simulink model "dsp_blr_hikaku_nakamura_futagi"  (R2018a)
settings: Solver=VariableStepAuto  StartTime=0.0  StopTime=100e-6  RelTol=1e-3
values from neighbouring files (symbols this model uses):
  BASELINE = 0    [dsp_blr.mat]
libraries: xbsIndex_r4 x934, xrbsSSR_Library x35, simulink x3, dspsigattribs x2, hdlsllib x2
(part 4 of 6)

== system dsp_blr_hikaku_nakamura_futagi/8sample_average 1/Vector_sum ==
  tdata_in : Inport
  AddSub{,1..3} (4 alike) : xbsIndex_r4/AddSub  mode=Addition  use_carryin=off  use_carryout=off  en=off  latency=0  precision=User Defined  arith_type="Signed  (2's comp)"  n_bits=17  bin_pt=4  quantization=Truncate  overflow=Wrap  use_behavioral_HDL=off  hw_selection=Fabric  pipelined=off  dbl_ovrd=off  block_type=addsub
  AddSub4 : xbsIndex_r4/AddSub  mode=Addition  use_carryin=off  use_carryout=off  en=off  latency=0  precision=Full  arith_type="Signed  (2's comp)"  n_bits=18  bin_pt=4  quantization=Truncate  overflow=Wrap  use_behavioral_HDL=off  hw_selection=Fabric  pipelined=off  dbl_ovrd=off  block_type=addsub
  AddSub5 : xbsIndex_r4/AddSub  mode=Addition  use_carryin=off  use_carryout=off  en=off  latency=0  precision=Full  arith_type="Signed  (2's comp)"  n_bits=18  bin_pt=4  quantization=Truncate  overflow=Wrap  use_behavioral_HDL=off  hw_selection=Fabric  pipelined=off  dbl_ovrd=off  block_type=addsub
  AddSub6 : xbsIndex_r4/AddSub  mode=Addition  use_carryin=off  use_carryout=off  en=off  latency=0  precision=User Defined  arith_type="Signed  (2's comp)"  n_bits=19  bin_pt=4  quantization=Truncate  overflow=Wrap  use_behavioral_HDL=off  hw_selection=Fabric  pipelined=off  dbl_ovrd=off  block_type=addsub
  Reinterpret{,1..7} (8 alike) : xbsIndex_r4/Reinterpret  force_arith_type=on  arith_type="Signed  (2's comp)"  force_bin_pt=on  bin_pt=4  block_type=reinterpret
  Slice : xbsIndex_r4/Slice  nbits=16  boolean_output=off  mode=Two Bit Locations  bit1=15  base1=LSB of Input  bit0=0  base0=LSB of Input  dbl_ovrd=off  block_type=slice
  Slice1 : xbsIndex_r4/Slice  nbits=16  boolean_output=off  mode=Two Bit Locations  bit1=31  base1=LSB of Input  bit0=16  base0=LSB of Input  dbl_ovrd=off  block_type=slice
  Slice2 : xbsIndex_r4/Slice  nbits=16  boolean_output=off  mode=Two Bit Locations  bit1=47  base1=LSB of Input  bit0=32  base0=LSB of Input  dbl_ovrd=off  block_type=slice
  Slice3 : xbsIndex_r4/Slice  nbits=16  boolean_output=off  mode=Two Bit Locations  bit1=63  base1=LSB of Input  bit0=48  base0=LSB of Input  dbl_ovrd=off  block_type=slice
  Slice4 : xbsIndex_r4/Slice  nbits=16  boolean_output=off  mode=Two Bit Locations  bit1=79  base1=LSB of Input  bit0=64  base0=LSB of Input  dbl_ovrd=off  block_type=slice
  Slice5 : xbsIndex_r4/Slice  nbits=16  boolean_output=off  mode=Two Bit Locations  bit1=95  base1=LSB of Input  bit0=80  base0=LSB of Input  dbl_ovrd=off  block_type=slice
  Slice6 : xbsIndex_r4/Slice  nbits=16  boolean_output=off  mode=Two Bit Locations  bit1=111  base1=LSB of Input  bit0=96  base0=LSB of Input  dbl_ovrd=off  block_type=slice
  Slice7 : xbsIndex_r4/Slice  nbits=16  boolean_output=off  mode=Two Bit Locations  bit1=127  base1=LSB of Input  bit0=112  base0=LSB of Input  dbl_ovrd=off  block_type=slice
  Vector Reinterpret : xrbsSSR_Library/Vector Reinterpret  sg_ssr=8  sg_ssr_prev=8  force_arith_type=on  arith_type=Unsigned  force_bin_pt=on  bin_pt=0  block_type=reinterpret_ssr
      settings: SourceProductName=Xilinx SSR Blockset  infoedit="The Vector Reinterpret block Changes vector input signal type without altering the binary representation. You can change the signal between signed and unsigned, and relocate the binary point.<br><br>Hardware notes: In hardware this block costs nothing.<br><br>Example:  Suppose the input is 6 bits wide, signed, with 2 fractional bits, and the output is forced to unsigned with 0 fractional bits.  Then an input of -2.0 (1110.00 in binary 2's complement) becomes an output of 56 (111000 in binary)."
  Vector2Scalar : xrbsSSR_Library/Vector2Scalar  sg_ssr=8  sg_ssr_prev=8  sg_ssr_name=vect_Vector2Scalar  block_type=vector2scalar_ssr
      settings: SourceProductName=Xilinx SSR Blockset
  sum_data_out : Outport  OutDataTypeStr=fixdt(1,19,4)
  wires:
  AddSub4/1 -> AddSub6/1
  Vector2Scalar/1 -> Slice7/1, Slice6/1, Slice5/1, Slice4/1, Slice2/1, Slice/1, Slice1/1, Slice3/1
  AddSub1/1 -> AddSub4/2
  AddSub5/1 -> AddSub6/2
  AddSub/1 -> AddSub4/1
  AddSub3/1 -> AddSub5/2
  AddSub2/1 -> AddSub5/1
  AddSub6/1 -> sum_data_out/1
  Slice/1 -> Reinterpret/1
  Slice1/1 -> Reinterpret1/1
  Slice2/1 -> Reinterpret2/1
  Slice3/1 -> Reinterpret3/1
  Slice4/1 -> Reinterpret4/1
  Slice5/1 -> Reinterpret5/1
  Slice6/1 -> Reinterpret6/1
  Slice7/1 -> Reinterpret7/1
  Reinterpret/1 -> AddSub/1
  Reinterpret1/1 -> AddSub/2
  Reinterpret2/1 -> AddSub1/1
  Reinterpret3/1 -> AddSub1/2
  Reinterpret4/1 -> AddSub2/1
  Reinterpret5/1 -> AddSub2/2
  Reinterpret6/1 -> AddSub3/1
  Reinterpret7/1 -> AddSub3/2
  tdata_in/1 -> Vector Reinterpret/1
  Vector Reinterpret/1 -> Vector2Scalar/1

== system dsp_blr_hikaku_nakamura_futagi/8sample_average 1/scaling ==
  valid_in : Inport
  data_in : Inport  Port=2
  Shift : xbsIndex_r4/Shift  shift_dir=Right  shift_bits=3  en=off  latency=1  precision=Full  arith_type="Signed  (2's comp)"  n_bits=16  bin_pt=14  quantization=Truncate  overflow=Wrap  dbl_ovrd=off  block_type=shift
  tvalid_delay : xbsIndex_r4/Delay  rst=off  infoeditControl=Selection of Reset will increase slice count due to use of real FFs and instead of SRLs  en=off  latency=1  reg_retiming=off  dbl_ovrd=off  block_type=delay
  valid_out : Outport
  data_out : Outport  Port=2
  wires:
  valid_in/1 -> tvalid_delay/1
  tvalid_delay/1 -> valid_out/1
  data_in/1 -> Shift/1
  Shift/1 -> data_out/1

== system dsp_blr_hikaku_nakamura_futagi/8sample_average 3/Vector_sum ==
  tdata_in : Inport
  AddSub{,1..3} (4 alike) : xbsIndex_r4/AddSub  mode=Addition  use_carryin=off  use_carryout=off  en=off  latency=0  precision=User Defined  arith_type="Signed  (2's comp)"  n_bits=17  bin_pt=4  quantization=Truncate  overflow=Wrap  use_behavioral_HDL=off  hw_selection=Fabric  pipelined=off  dbl_ovrd=off  block_type=addsub
  AddSub4 : xbsIndex_r4/AddSub  mode=Addition  use_carryin=off  use_carryout=off  en=off  latency=0  precision=Full  arith_type="Signed  (2's comp)"  n_bits=18  bin_pt=4  quantization=Truncate  overflow=Wrap  use_behavioral_HDL=off  hw_selection=Fabric  pipelined=off  dbl_ovrd=off  block_type=addsub
  AddSub5 : xbsIndex_r4/AddSub  mode=Addition  use_carryin=off  use_carryout=off  en=off  latency=0  precision=Full  arith_type="Signed  (2's comp)"  n_bits=18  bin_pt=4  quantization=Truncate  overflow=Wrap  use_behavioral_HDL=off  hw_selection=Fabric  pipelined=off  dbl_ovrd=off  block_type=addsub
  AddSub6 : xbsIndex_r4/AddSub  mode=Addition  use_carryin=off  use_carryout=off  en=off  latency=0  precision=User Defined  arith_type="Signed  (2's comp)"  n_bits=19  bin_pt=4  quantization=Truncate  overflow=Wrap  use_behavioral_HDL=off  hw_selection=Fabric  pipelined=off  dbl_ovrd=off  block_type=addsub
  Gateway Out6 : xbsIndex_r4/Gateway Out  inherit_from_input=off  hdl_port=on  rows=1  columns=1  UseAsDAC=off  DACChannel='1'  interface=None  automatic_assignment=on  address_offset=hex2dec('00')  intf_name=''  intf_description=''  timing_constraint=None  locs_specified=off  LOCs={}  io_standard={}  block_type=gatewayout
  Reinterpret{,1..7} (8 alike) : xbsIndex_r4/Reinterpret  force_arith_type=on  arith_type="Signed  (2's comp)"  force_bin_pt=on  bin_pt=4  block_type=reinterpret
  Scope8 : Scope  NumInputPorts=2
  Slice : xbsIndex_r4/Slice  nbits=16  boolean_output=off  mode=Two Bit Locations  bit1=15  base1=LSB of Input  bit0=0  base0=LSB of Input  dbl_ovrd=off  block_type=slice
  Slice1 : xbsIndex_r4/Slice  nbits=16  boolean_output=off  mode=Two Bit Locations  bit1=31  base1=LSB of Input  bit0=16  base0=LSB of Input  dbl_ovrd=off  block_type=slice
  Slice2 : xbsIndex_r4/Slice  nbits=16  boolean_output=off  mode=Two Bit Locations  bit1=47  base1=LSB of Input  bit0=32  base0=LSB of Input  dbl_ovrd=off  block_type=slice
  Slice3 : xbsIndex_r4/Slice  nbits=16  boolean_output=off  mode=Two Bit Locations  bit1=63  base1=LSB of Input  bit0=48  base0=LSB of Input  dbl_ovrd=off  block_type=slice
  Slice4 : xbsIndex_r4/Slice  nbits=16  boolean_output=off  mode=Two Bit Locations  bit1=79  base1=LSB of Input  bit0=64  base0=LSB of Input  dbl_ovrd=off  block_type=slice
  Slice5 : xbsIndex_r4/Slice  nbits=16  boolean_output=off  mode=Two Bit Locations  bit1=95  base1=LSB of Input  bit0=80  base0=LSB of Input  dbl_ovrd=off  block_type=slice
  Slice6 : xbsIndex_r4/Slice  nbits=16  boolean_output=off  mode=Two Bit Locations  bit1=111  base1=LSB of Input  bit0=96  base0=LSB of Input  dbl_ovrd=off  block_type=slice
  Slice7 : xbsIndex_r4/Slice  nbits=16  boolean_output=off  mode=Two Bit Locations  bit1=127  base1=LSB of Input  bit0=112  base0=LSB of Input  dbl_ovrd=off  block_type=slice
  Vector Real Gateway Out1 : xrbsSSR_Library/Vector Real Gateway Out  inherit_from_input=off  hdl_port=on  rows=1  columns=1  UseAsDAC=off  DACChannel='1'  interface=None  automatic_assignment=on  address_offset=hex2dec('00')  intf_name=''  intf_description=''  timing_constraint=None  locs_specified=off  LOCs={}  io_standard={}  block_type=realgatewayout_ssr  sg_ssr=8  sg_ssr_prev=8  sg_ssr_name=vect_real_gwayout
      settings: SourceProductName=Xilinx SSR Blockset  infoedit=The Vector Real Gateway out block converts Xilinx fixed-point or floating-point type vector inputs into vector ouputs of type Simulink integer, single, double, or fixed-point.<br><br>Hardware notes: In hardware these blocks become top level output ports or are discarded, depending on how they are configured.
  Vector Reinterpret : xrbsSSR_Library/Vector Reinterpret  sg_ssr=8  sg_ssr_prev=8  force_arith_type=on  arith_type=Unsigned  force_bin_pt=on  bin_pt=0  block_type=reinterpret_ssr
      settings: SourceProductName=Xilinx SSR Blockset  infoedit="The Vector Reinterpret block Changes vector input signal type without altering the binary representation. You can change the signal between signed and unsigned, and relocate the binary point.<br><br>Hardware notes: In hardware this block costs nothing.<br><br>Example:  Suppose the input is 6 bits wide, signed, with 2 fractional bits, and the output is forced to unsigned with 0 fractional bits.  Then an input of -2.0 (1110.00 in binary 2's complement) becomes an output of 56 (111000 in binary)."
  Vector2Scalar : xrbsSSR_Library/Vector2Scalar  sg_ssr=8  sg_ssr_prev=8  sg_ssr_name=vect_Vector2Scalar  block_type=vector2scalar_ssr
      settings: SourceProductName=Xilinx SSR Blockset
  sum_data_out : Outport  OutDataTypeStr=fixdt(1,19,4)
  wires:
  AddSub4/1 -> AddSub6/1
  Vector2Scalar/1 -> Slice7/1, Slice6/1, Slice5/1, Slice4/1, Slice2/1, Slice/1, Slice1/1, Slice3/1
  AddSub1/1 -> AddSub4/2
  AddSub5/1 -> AddSub6/2
  AddSub/1 -> AddSub4/1
  AddSub3/1 -> AddSub5/2
  AddSub2/1 -> AddSub5/1
  AddSub6/1 -> Gateway Out6/1, sum_data_out/1
  Slice/1 -> Reinterpret/1
  Slice1/1 -> Reinterpret1/1
  Slice2/1 -> Reinterpret2/1
  Slice3/1 -> Reinterpret3/1
  Slice4/1 -> Reinterpret4/1
  Slice5/1 -> Reinterpret5/1
  Slice6/1 -> Reinterpret6/1
  Slice7/1 -> Reinterpret7/1
  Reinterpret/1 -> AddSub/1
  Reinterpret1/1 -> AddSub/2
  Reinterpret2/1 -> AddSub1/1
  Reinterpret3/1 -> AddSub1/2
  Reinterpret4/1 -> AddSub2/1
  Reinterpret5/1 -> AddSub2/2
  Reinterpret6/1 -> AddSub3/1
  Reinterpret7/1 -> AddSub3/2
  tdata_in/1 -> Vector Real Gateway Out1/1, Vector Reinterpret/1
  Vector Reinterpret/1 -> Vector2Scalar/1
  Gateway Out6/1 -> Scope8/2  "scalar"
  Vector Real Gateway Out1/1 -> Scope8/1  "vector"

== system dsp_blr_hikaku_nakamura_futagi/8sample_average 3/scaling ==
  valid_in : Inport
  data_in : Inport  Port=2
  Gateway Out1 : xbsIndex_r4/Gateway Out  inherit_from_input=off  hdl_port=on  rows=1  columns=1  UseAsDAC=off  DACChannel='1'  interface=None  automatic_assignment=on  address_offset=hex2dec('00')  intf_name=''  intf_description=''  timing_constraint=None  locs_specified=off  LOCs={}  io_standard={}  block_type=gatewayout
  Gateway Out6 : xbsIndex_r4/Gateway Out  inherit_from_input=off  hdl_port=on  rows=1  columns=1  UseAsDAC=off  DACChannel='1'  interface=None  automatic_assignment=on  address_offset=hex2dec('00')  intf_name=''  intf_description=''  timing_constraint=None  locs_specified=off  LOCs={}  io_standard={}  block_type=gatewayout
  Scope8 : Scope  NumInputPorts=2
  Shift : xbsIndex_r4/Shift  shift_dir=Right  shift_bits=3  en=off  latency=1  precision=Full  arith_type="Signed  (2's comp)"  n_bits=16  bin_pt=14  quantization=Truncate  overflow=Wrap  dbl_ovrd=off  block_type=shift
  tvalid_delay : xbsIndex_r4/Delay  rst=off  infoeditControl=Selection of Reset will increase slice count due to use of real FFs and instead of SRLs  en=off  latency=1  reg_retiming=off  dbl_ovrd=off  block_type=delay
  valid_out : Outport
  data_out : Outport  Port=2
  wires:
  valid_in/1 -> tvalid_delay/1
  tvalid_delay/1 -> valid_out/1
  data_in/1 -> Gateway Out1/1, Shift/1
  Gateway Out6/1 -> Scope8/2  "after"
  Gateway Out1/1 -> Scope8/1  "before"
  Shift/1 -> Gateway Out6/1, data_out/1

== system dsp_blr_hikaku_nakamura_futagi/Ave10/Subsystem1 ==
  In1 : Inport
  AddSub{,1,3,8..9,12} (6 alike) : xbsIndex_r4/AddSub  mode=Addition  use_carryin=off  use_carryout=off  en=off  latency=0  precision=User Defined  arith_type="Signed  (2's comp)"  n_bits=17  bin_pt=4  quantization=Truncate  overflow=Wrap  use_behavioral_HDL=off  hw_selection=Fabric  pipelined=off  dbl_ovrd=off  block_type=addsub
  AddSub4 : xbsIndex_r4/AddSub  mode=Addition  use_carryin=off  use_carryout=off  en=off  latency=0  precision=Full  arith_type="Signed  (2's comp)"  n_bits=18  bin_pt=4  quantization=Truncate  overflow=Wrap  use_behavioral_HDL=off  hw_selection=Fabric  pipelined=off  dbl_ovrd=off  block_type=addsub
  Delay1 : xbsIndex_r4/Delay  rst=off  infoeditControl=Selection of Reset will increase slice count due to use of real FFs and instead of SRLs  en=off  latency=1  reg_retiming=off  dbl_ovrd=off  block_type=delay
  Delay10 : xbsIndex_r4/Delay  rst=off  infoeditControl=Selection of Reset will increase slice count due to use of real FFs and instead of SRLs  en=off  latency=7  reg_retiming=off  dbl_ovrd=off  block_type=delay
  Delay2 : xbsIndex_r4/Delay  rst=off  infoeditControl=Selection of Reset will increase slice count due to use of real FFs and instead of SRLs  en=off  latency=2  reg_retiming=off  dbl_ovrd=off  block_type=delay
  Delay5 : xbsIndex_r4/Delay  rst=off  infoeditControl=Selection of Reset will increase slice count due to use of real FFs and instead of SRLs  en=off  latency=3  reg_retiming=off  dbl_ovrd=off  block_type=delay
  Delay7 : xbsIndex_r4/Delay  rst=off  infoeditControl=Selection of Reset will increase slice count due to use of real FFs and instead of SRLs  en=off  latency=4  reg_retiming=off  dbl_ovrd=off  block_type=delay
  Delay8 : xbsIndex_r4/Delay  rst=off  infoeditControl=Selection of Reset will increase slice count due to use of real FFs and instead of SRLs  en=off  latency=5  reg_retiming=off  dbl_ovrd=off  block_type=delay
  Delay9 : xbsIndex_r4/Delay  rst=off  infoeditControl=Selection of Reset will increase slice count due to use of real FFs and instead of SRLs  en=off  latency=6  reg_retiming=off  dbl_ovrd=off  block_type=delay
  Out1 : Outport
  wires:
  AddSub/1 -> AddSub1/1
  In1/1 -> AddSub/1, Delay10/1, Delay9/1, Delay8/1, Delay7/1, Delay5/1, Delay2/1, Delay1/1
  AddSub9/1 -> AddSub12/2
  Delay1/1 -> AddSub/2
  Delay10/1 -> AddSub9/2
  Delay9/1 -> AddSub9/1
  Delay2/1 -> AddSub3/1
  AddSub4/1 -> Out1/1
  Delay7/1 -> AddSub8/1
  AddSub1/1 -> AddSub4/1
  Delay8/1 -> AddSub8/2
  AddSub8/1 -> AddSub12/1
  Delay5/1 -> AddSub3/2
  AddSub3/1 -> AddSub1/2
  AddSub12/1 -> AddSub4/2

== system dsp_blr_hikaku_nakamura_futagi/Ave10/Subsystem2 ==
  In1 : Inport
  AddSub{,1,3,8..9,12} (6 alike) : xbsIndex_r4/AddSub  mode=Addition  use_carryin=off  use_carryout=off  en=off  latency=0  precision=User Defined  arith_type="Signed  (2's comp)"  n_bits=17  bin_pt=4  quantization=Truncate  overflow=Wrap  use_behavioral_HDL=off  hw_selection=Fabric  pipelined=off  dbl_ovrd=off  block_type=addsub
  AddSub4 : xbsIndex_r4/AddSub  mode=Addition  use_carryin=off  use_carryout=off  en=off  latency=0  precision=Full  arith_type="Signed  (2's comp)"  n_bits=18  bin_pt=4  quantization=Truncate  overflow=Wrap  use_behavioral_HDL=off  hw_selection=Fabric  pipelined=off  dbl_ovrd=off  block_type=addsub
  Delay1 : xbsIndex_r4/Delay  rst=off  infoeditControl=Selection of Reset will increase slice count due to use of real FFs and instead of SRLs  en=off  latency=1  reg_retiming=off  dbl_ovrd=off  block_type=delay
  Delay10 : xbsIndex_r4/Delay  rst=off  infoeditControl=Selection of Reset will increase slice count due to use of real FFs and instead of SRLs  en=off  latency=7  reg_retiming=off  dbl_ovrd=off  block_type=delay
  Delay2 : xbsIndex_r4/Delay  rst=off  infoeditControl=Selection of Reset will increase slice count due to use of real FFs and instead of SRLs  en=off  latency=2  reg_retiming=off  dbl_ovrd=off  block_type=delay
  Delay5 : xbsIndex_r4/Delay  rst=off  infoeditControl=Selection of Reset will increase slice count due to use of real FFs and instead of SRLs  en=off  latency=3  reg_retiming=off  dbl_ovrd=off  block_type=delay
  Delay7 : xbsIndex_r4/Delay  rst=off  infoeditControl=Selection of Reset will increase slice count due to use of real FFs and instead of SRLs  en=off  latency=4  reg_retiming=off  dbl_ovrd=off  block_type=delay
  Delay8 : xbsIndex_r4/Delay  rst=off  infoeditControl=Selection of Reset will increase slice count due to use of real FFs and instead of SRLs  en=off  latency=5  reg_retiming=off  dbl_ovrd=off  block_type=delay
  Delay9 : xbsIndex_r4/Delay  rst=off  infoeditControl=Selection of Reset will increase slice count due to use of real FFs and instead of SRLs  en=off  latency=6  reg_retiming=off  dbl_ovrd=off  block_type=delay
  Out1 : Outport
  wires:
  AddSub/1 -> AddSub1/1
  In1/1 -> AddSub/1, Delay10/1, Delay9/1, Delay8/1, Delay7/1, Delay5/1, Delay2/1, Delay1/1
  AddSub9/1 -> AddSub12/2
  Delay1/1 -> AddSub/2
  Delay10/1 -> AddSub9/2
  Delay9/1 -> AddSub9/1
  Delay2/1 -> AddSub3/1
  AddSub4/1 -> Out1/1
  Delay7/1 -> AddSub8/1
  AddSub1/1 -> AddSub4/1
  Delay8/1 -> AddSub8/2
  AddSub8/1 -> AddSub12/1
  Delay5/1 -> AddSub3/2
  AddSub3/1 -> AddSub1/2
  AddSub12/1 -> AddSub4/2

== system dsp_blr_hikaku_nakamura_futagi/Ave10/Subsystem3 ==
  In1 : Inport
  AddSub{,1,3,8..9,12} (6 alike) : xbsIndex_r4/AddSub  mode=Addition  use_carryin=off  use_carryout=off  en=off  latency=0  precision=User Defined  arith_type="Signed  (2's comp)"  n_bits=17  bin_pt=4  quantization=Truncate  overflow=Wrap  use_behavioral_HDL=off  hw_selection=Fabric  pipelined=off  dbl_ovrd=off  block_type=addsub
  AddSub4 : xbsIndex_r4/AddSub  mode=Addition  use_carryin=off  use_carryout=off  en=off  latency=0  precision=Full  arith_type="Signed  (2's comp)"  n_bits=18  bin_pt=4  quantization=Truncate  overflow=Wrap  use_behavioral_HDL=off  hw_selection=Fabric  pipelined=off  dbl_ovrd=off  block_type=addsub
  Delay1 : xbsIndex_r4/Delay  rst=off  infoeditControl=Selection of Reset will increase slice count due to use of real FFs and instead of SRLs  en=off  latency=1  reg_retiming=off  dbl_ovrd=off  block_type=delay
  Delay10 : xbsIndex_r4/Delay  rst=off  infoeditControl=Selection of Reset will increase slice count due to use of real FFs and instead of SRLs  en=off  latency=7  reg_retiming=off  dbl_ovrd=off  block_type=delay
  Delay2 : xbsIndex_r4/Delay  rst=off  infoeditControl=Selection of Reset will increase slice count due to use of real FFs and instead of SRLs  en=off  latency=2  reg_retiming=off  dbl_ovrd=off  block_type=delay
  Delay5 : xbsIndex_r4/Delay  rst=off  infoeditControl=Selection of Reset will increase slice count due to use of real FFs and instead of SRLs  en=off  latency=3  reg_retiming=off  dbl_ovrd=off  block_type=delay
  Delay7 : xbsIndex_r4/Delay  rst=off  infoeditControl=Selection of Reset will increase slice count due to use of real FFs and instead of SRLs  en=off  latency=4  reg_retiming=off  dbl_ovrd=off  block_type=delay
  Delay8 : xbsIndex_r4/Delay  rst=off  infoeditControl=Selection of Reset will increase slice count due to use of real FFs and instead of SRLs  en=off  latency=5  reg_retiming=off  dbl_ovrd=off  block_type=delay
  Delay9 : xbsIndex_r4/Delay  rst=off  infoeditControl=Selection of Reset will increase slice count due to use of real FFs and instead of SRLs  en=off  latency=6  reg_retiming=off  dbl_ovrd=off  block_type=delay
  Out1 : Outport
  wires:
  AddSub/1 -> AddSub1/1
  In1/1 -> AddSub/1, Delay10/1, Delay9/1, Delay8/1, Delay7/1, Delay5/1, Delay2/1, Delay1/1
  AddSub9/1 -> AddSub12/2
  Delay1/1 -> AddSub/2
  Delay10/1 -> AddSub9/2
  Delay9/1 -> AddSub9/1
  Delay2/1 -> AddSub3/1
  AddSub4/1 -> Out1/1
  Delay7/1 -> AddSub8/1
  AddSub1/1 -> AddSub4/1
  Delay8/1 -> AddSub8/2
  AddSub8/1 -> AddSub12/1
  Delay5/1 -> AddSub3/2
  AddSub3/1 -> AddSub1/2
  AddSub12/1 -> AddSub4/2

== system dsp_blr_hikaku_nakamura_futagi/Ave10/Subsystem4 ==
  In1 : Inport
  AddSub{,1,3,8..9,12} (6 alike) : xbsIndex_r4/AddSub  mode=Addition  use_carryin=off  use_carryout=off  en=off  latency=0  precision=User Defined  arith_type="Signed  (2's comp)"  n_bits=17  bin_pt=4  quantization=Truncate  overflow=Wrap  use_behavioral_HDL=off  hw_selection=Fabric  pipelined=off  dbl_ovrd=off  block_type=addsub
  AddSub4 : xbsIndex_r4/AddSub  mode=Addition  use_carryin=off  use_carryout=off  en=off  latency=0  precision=Full  arith_type="Signed  (2's comp)"  n_bits=18  bin_pt=4  quantization=Truncate  overflow=Wrap  use_behavioral_HDL=off  hw_selection=Fabric  pipelined=off  dbl_ovrd=off  block_type=addsub
  Delay1 : xbsIndex_r4/Delay  rst=off  infoeditControl=Selection of Reset will increase slice count due to use of real FFs and instead of SRLs  en=off  latency=1  reg_retiming=off  dbl_ovrd=off  block_type=delay
  Delay10 : xbsIndex_r4/Delay  rst=off  infoeditControl=Selection of Reset will increase slice count due to use of real FFs and instead of SRLs  en=off  latency=7  reg_retiming=off  dbl_ovrd=off  block_type=delay
  Delay2 : xbsIndex_r4/Delay  rst=off  infoeditControl=Selection of Reset will increase slice count due to use of real FFs and instead of SRLs  en=off  latency=2  reg_retiming=off  dbl_ovrd=off  block_type=delay
  Delay5 : xbsIndex_r4/Delay  rst=off  infoeditControl=Selection of Reset will increase slice count due to use of real FFs and instead of SRLs  en=off  latency=3  reg_retiming=off  dbl_ovrd=off  block_type=delay
  Delay7 : xbsIndex_r4/Delay  rst=off  infoeditControl=Selection of Reset will increase slice count due to use of real FFs and instead of SRLs  en=off  latency=4  reg_retiming=off  dbl_ovrd=off  block_type=delay
  Delay8 : xbsIndex_r4/Delay  rst=off  infoeditControl=Selection of Reset will increase slice count due to use of real FFs and instead of SRLs  en=off  latency=5  reg_retiming=off  dbl_ovrd=off  block_type=delay
  Delay9 : xbsIndex_r4/Delay  rst=off  infoeditControl=Selection of Reset will increase slice count due to use of real FFs and instead of SRLs  en=off  latency=6  reg_retiming=off  dbl_ovrd=off  block_type=delay
  Out1 : Outport
  wires:
  AddSub/1 -> AddSub1/1
  In1/1 -> AddSub/1, Delay10/1, Delay9/1, Delay8/1, Delay7/1, Delay5/1, Delay2/1, Delay1/1
  AddSub9/1 -> AddSub12/2
  Delay1/1 -> AddSub/2
  Delay10/1 -> AddSub9/2
  Delay9/1 -> AddSub9/1
  Delay2/1 -> AddSub3/1
  AddSub4/1 -> Out1/1
  Delay7/1 -> AddSub8/1
  AddSub1/1 -> AddSub4/1
  Delay8/1 -> AddSub8/2
  AddSub8/1 -> AddSub12/1
  Delay5/1 -> AddSub3/2
  AddSub3/1 -> AddSub1/2
  AddSub12/1 -> AddSub4/2

== system dsp_blr_hikaku_nakamura_futagi/Ave10/Subsystem5 ==
  In1 : Inport
  AddSub{,1,3,8..9,12} (6 alike) : xbsIndex_r4/AddSub  mode=Addition  use_carryin=off  use_carryout=off  en=off  latency=0  precision=User Defined  arith_type="Signed  (2's comp)"  n_bits=17  bin_pt=4  quantization=Truncate  overflow=Wrap  use_behavioral_HDL=off  hw_selection=Fabric  pipelined=off  dbl_ovrd=off  block_type=addsub
  AddSub4 : xbsIndex_r4/AddSub  mode=Addition  use_carryin=off  use_carryout=off  en=off  latency=0  precision=Full  arith_type="Signed  (2's comp)"  n_bits=18  bin_pt=4  quantization=Truncate  overflow=Wrap  use_behavioral_HDL=off  hw_selection=Fabric  pipelined=off  dbl_ovrd=off  block_type=addsub
  Delay1 : xbsIndex_r4/Delay  rst=off  infoeditControl=Selection of Reset will increase slice count due to use of real FFs and instead of SRLs  en=off  latency=1  reg_retiming=off  dbl_ovrd=off  block_type=delay
  Delay10 : xbsIndex_r4/Delay  rst=off  infoeditControl=Selection of Reset will increase slice count due to use of real FFs and instead of SRLs  en=off  latency=7  reg_retiming=off  dbl_ovrd=off  block_type=delay
  Delay2 : xbsIndex_r4/Delay  rst=off  infoeditControl=Selection of Reset will increase slice count due to use of real FFs and instead of SRLs  en=off  latency=2  reg_retiming=off  dbl_ovrd=off  block_type=delay
  Delay5 : xbsIndex_r4/Delay  rst=off  infoeditControl=Selection of Reset will increase slice count due to use of real FFs and instead of SRLs  en=off  latency=3  reg_retiming=off  dbl_ovrd=off  block_type=delay
  Delay7 : xbsIndex_r4/Delay  rst=off  infoeditControl=Selection of Reset will increase slice count due to use of real FFs and instead of SRLs  en=off  latency=4  reg_retiming=off  dbl_ovrd=off  block_type=delay
  Delay8 : xbsIndex_r4/Delay  rst=off  infoeditControl=Selection of Reset will increase slice count due to use of real FFs and instead of SRLs  en=off  latency=5  reg_retiming=off  dbl_ovrd=off  block_type=delay
  Delay9 : xbsIndex_r4/Delay  rst=off  infoeditControl=Selection of Reset will increase slice count due to use of real FFs and instead of SRLs  en=off  latency=6  reg_retiming=off  dbl_ovrd=off  block_type=delay
  Out1 : Outport
  wires:
  AddSub/1 -> AddSub1/1
  In1/1 -> AddSub/1, Delay10/1, Delay9/1, Delay8/1, Delay7/1, Delay5/1, Delay2/1, Delay1/1
  AddSub9/1 -> AddSub12/2
  Delay1/1 -> AddSub/2
  Delay10/1 -> AddSub9/2
  Delay9/1 -> AddSub9/1
  Delay2/1 -> AddSub3/1
  AddSub4/1 -> Out1/1
  Delay7/1 -> AddSub8/1
  AddSub1/1 -> AddSub4/1
  Delay8/1 -> AddSub8/2
  AddSub8/1 -> AddSub12/1
  Delay5/1 -> AddSub3/2
  AddSub3/1 -> AddSub1/2
  AddSub12/1 -> AddSub4/2

== system dsp_blr_hikaku_nakamura_futagi/Ave10/Subsystem6 ==
  In1 : Inport
  AddSub{,1,3,8..9,12} (6 alike) : xbsIndex_r4/AddSub  mode=Addition  use_carryin=off  use_carryout=off  en=off  latency=0  precision=User Defined  arith_type="Signed  (2's comp)"  n_bits=17  bin_pt=4  quantization=Truncate  overflow=Wrap  use_behavioral_HDL=off  hw_selection=Fabric  pipelined=off  dbl_ovrd=off  block_type=addsub
  AddSub4 : xbsIndex_r4/AddSub  mode=Addition  use_carryin=off  use_carryout=off  en=off  latency=0  precision=Full  arith_type="Signed  (2's comp)"  n_bits=18  bin_pt=4  quantization=Truncate  overflow=Wrap  use_behavioral_HDL=off  hw_selection=Fabric  pipelined=off  dbl_ovrd=off  block_type=addsub
  Delay1 : xbsIndex_r4/Delay  rst=off  infoeditControl=Selection of Reset will increase slice count due to use of real FFs and instead of SRLs  en=off  latency=1  reg_retiming=off  dbl_ovrd=off  block_type=delay
  Delay10 : xbsIndex_r4/Delay  rst=off  infoeditControl=Selection of Reset will increase slice count due to use of real FFs and instead of SRLs  en=off  latency=7  reg_retiming=off  dbl_ovrd=off  block_type=delay
  Delay2 : xbsIndex_r4/Delay  rst=off  infoeditControl=Selection of Reset will increase slice count due to use of real FFs and instead of SRLs  en=off  latency=2  reg_retiming=off  dbl_ovrd=off  block_type=delay
  Delay5 : xbsIndex_r4/Delay  rst=off  infoeditControl=Selection of Reset will increase slice count due to use of real FFs and instead of SRLs  en=off  latency=3  reg_retiming=off  dbl_ovrd=off  block_type=delay
  Delay7 : xbsIndex_r4/Delay  rst=off  infoeditControl=Selection of Reset will increase slice count due to use of real FFs and instead of SRLs  en=off  latency=4  reg_retiming=off  dbl_ovrd=off  block_type=delay
  Delay8 : xbsIndex_r4/Delay  rst=off  infoeditControl=Selection of Reset will increase slice count due to use of real FFs and instead of SRLs  en=off  latency=5  reg_retiming=off  dbl_ovrd=off  block_type=delay
  Delay9 : xbsIndex_r4/Delay  rst=off  infoeditControl=Selection of Reset will increase slice count due to use of real FFs and instead of SRLs  en=off  latency=6  reg_retiming=off  dbl_ovrd=off  block_type=delay
  Out1 : Outport
  wires:
  AddSub/1 -> AddSub1/1
  In1/1 -> AddSub/1, Delay10/1, Delay9/1, Delay8/1, Delay7/1, Delay5/1, Delay2/1, Delay1/1
  AddSub9/1 -> AddSub12/2
  Delay1/1 -> AddSub/2
  Delay10/1 -> AddSub9/2
  Delay9/1 -> AddSub9/1
  Delay2/1 -> AddSub3/1
  AddSub4/1 -> Out1/1
  Delay7/1 -> AddSub8/1
  AddSub1/1 -> AddSub4/1
  Delay8/1 -> AddSub8/2
  AddSub8/1 -> AddSub12/1
  Delay5/1 -> AddSub3/2
  AddSub3/1 -> AddSub1/2
  AddSub12/1 -> AddSub4/2

== system dsp_blr_hikaku_nakamura_futagi/Ave10/Subsystem7 ==
  In1 : Inport
  AddSub{,1,3,8..9,12} (6 alike) : xbsIndex_r4/AddSub  mode=Addition  use_carryin=off  use_carryout=off  en=off  latency=0  precision=User Defined  arith_type="Signed  (2's comp)"  n_bits=17  bin_pt=4  quantization=Truncate  overflow=Wrap  use_behavioral_HDL=off  hw_selection=Fabric  pipelined=off  dbl_ovrd=off  block_type=addsub
  AddSub4 : xbsIndex_r4/AddSub  mode=Addition  use_carryin=off  use_carryout=off  en=off  latency=0  precision=Full  arith_type="Signed  (2's comp)"  n_bits=18  bin_pt=4  quantization=Truncate  overflow=Wrap  use_behavioral_HDL=off  hw_selection=Fabric  pipelined=off  dbl_ovrd=off  block_type=addsub
  Delay1 : xbsIndex_r4/Delay  rst=off  infoeditControl=Selection of Reset will increase slice count due to use of real FFs and instead of SRLs  en=off  latency=1  reg_retiming=off  dbl_ovrd=off  block_type=delay
  Delay10 : xbsIndex_r4/Delay  rst=off  infoeditControl=Selection of Reset will increase slice count due to use of real FFs and instead of SRLs  en=off  latency=7  reg_retiming=off  dbl_ovrd=off  block_type=delay
  Delay2 : xbsIndex_r4/Delay  rst=off  infoeditControl=Selection of Reset will increase slice count due to use of real FFs and instead of SRLs  en=off  latency=2  reg_retiming=off  dbl_ovrd=off  block_type=delay
  Delay5 : xbsIndex_r4/Delay  rst=off  infoeditControl=Selection of Reset will increase slice count due to use of real FFs and instead of SRLs  en=off  latency=3  reg_retiming=off  dbl_ovrd=off  block_type=delay
  Delay7 : xbsIndex_r4/Delay  rst=off  infoeditControl=Selection of Reset will increase slice count due to use of real FFs and instead of SRLs  en=off  latency=4  reg_retiming=off  dbl_ovrd=off  block_type=delay
  Delay8 : xbsIndex_r4/Delay  rst=off  infoeditControl=Selection of Reset will increase slice count due to use of real FFs and instead of SRLs  en=off  latency=5  reg_retiming=off  dbl_ovrd=off  block_type=delay
  Delay9 : xbsIndex_r4/Delay  rst=off  infoeditControl=Selection of Reset will increase slice count due to use of real FFs and instead of SRLs  en=off  latency=6  reg_retiming=off  dbl_ovrd=off  block_type=delay
  Out1 : Outport
  wires:
  AddSub/1 -> AddSub1/1
  In1/1 -> AddSub/1, Delay10/1, Delay9/1, Delay8/1, Delay7/1, Delay5/1, Delay2/1, Delay1/1
  AddSub9/1 -> AddSub12/2
  Delay1/1 -> AddSub/2
  Delay10/1 -> AddSub9/2
  Delay9/1 -> AddSub9/1
  Delay2/1 -> AddSub3/1
  AddSub4/1 -> Out1/1
  Delay7/1 -> AddSub8/1
  AddSub1/1 -> AddSub4/1
  Delay8/1 -> AddSub8/2
  AddSub8/1 -> AddSub12/1
  Delay5/1 -> AddSub3/2
  AddSub3/1 -> AddSub1/2
  AddSub12/1 -> AddSub4/2

== system dsp_blr_hikaku_nakamura_futagi/Ave10/Subsystem8 ==
  In1 : Inport
  AddSub{,1,3,8..9,12} (6 alike) : xbsIndex_r4/AddSub  mode=Addition  use_carryin=off  use_carryout=off  en=off  latency=0  precision=User Defined  arith_type="Signed  (2's comp)"  n_bits=17  bin_pt=4  quantization=Truncate  overflow=Wrap  use_behavioral_HDL=off  hw_selection=Fabric  pipelined=off  dbl_ovrd=off  block_type=addsub
  AddSub4 : xbsIndex_r4/AddSub  mode=Addition  use_carryin=off  use_carryout=off  en=off  latency=0  precision=Full  arith_type="Signed  (2's comp)"  n_bits=18  bin_pt=4  quantization=Truncate  overflow=Wrap  use_behavioral_HDL=off  hw_selection=Fabric  pipelined=off  dbl_ovrd=off  block_type=addsub
  Delay1 : xbsIndex_r4/Delay  rst=off  infoeditControl=Selection of Reset will increase slice count due to use of real FFs and instead of SRLs  en=off  latency=1  reg_retiming=off  dbl_ovrd=off  block_type=delay
  Delay10 : xbsIndex_r4/Delay  rst=off  infoeditControl=Selection of Reset will increase slice count due to use of real FFs and instead of SRLs  en=off  latency=7  reg_retiming=off  dbl_ovrd=off  block_type=delay
  Delay2 : xbsIndex_r4/Delay  rst=off  infoeditControl=Selection of Reset will increase slice count due to use of real FFs and instead of SRLs  en=off  latency=2  reg_retiming=off  dbl_ovrd=off  block_type=delay
  Delay5 : xbsIndex_r4/Delay  rst=off  infoeditControl=Selection of Reset will increase slice count due to use of real FFs and instead of SRLs  en=off  latency=3  reg_retiming=off  dbl_ovrd=off  block_type=delay
  Delay7 : xbsIndex_r4/Delay  rst=off  infoeditControl=Selection of Reset will increase slice count due to use of real FFs and instead of SRLs  en=off  latency=4  reg_retiming=off  dbl_ovrd=off  block_type=delay
  Delay8 : xbsIndex_r4/Delay  rst=off  infoeditControl=Selection of Reset will increase slice count due to use of real FFs and instead of SRLs  en=off  latency=5  reg_retiming=off  dbl_ovrd=off  block_type=delay
  Delay9 : xbsIndex_r4/Delay  rst=off  infoeditControl=Selection of Reset will increase slice count due to use of real FFs and instead of SRLs  en=off  latency=6  reg_retiming=off  dbl_ovrd=off  block_type=delay
  Out1 : Outport
  wires:
  AddSub/1 -> AddSub1/1
  In1/1 -> AddSub/1, Delay10/1, Delay9/1, Delay8/1, Delay7/1, Delay5/1, Delay2/1, Delay1/1
  AddSub9/1 -> AddSub12/2
  Delay1/1 -> AddSub/2
  Delay10/1 -> AddSub9/2
  Delay9/1 -> AddSub9/1
  Delay2/1 -> AddSub3/1
  AddSub4/1 -> Out1/1
  Delay7/1 -> AddSub8/1
  AddSub1/1 -> AddSub4/1
  Delay8/1 -> AddSub8/2
  AddSub8/1 -> AddSub12/1
  Delay5/1 -> AddSub3/2
  AddSub3/1 -> AddSub1/2
  AddSub12/1 -> AddSub4/2

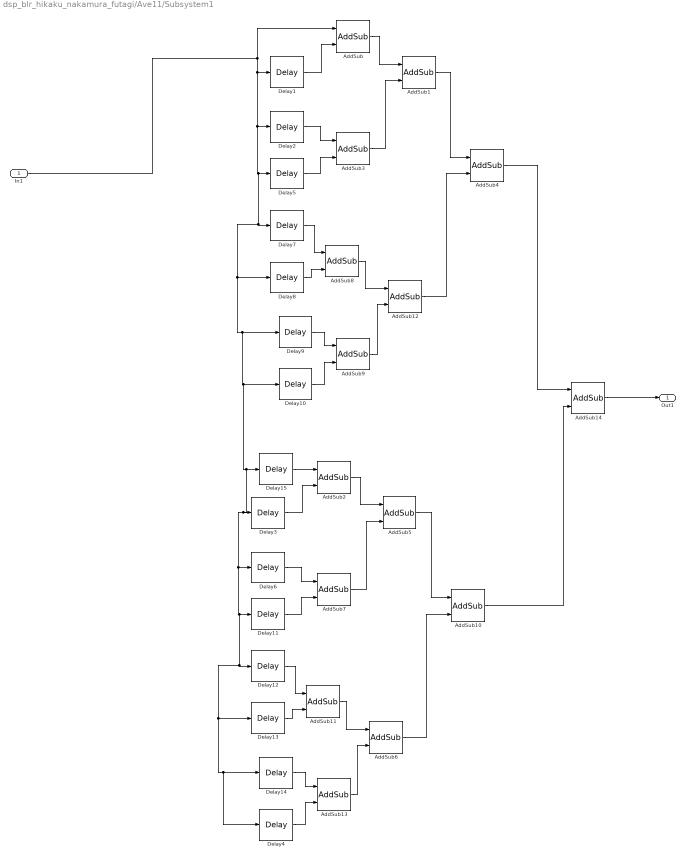
== system dsp_blr_hikaku_nakamura_futagi/Ave11/Subsystem1 ==
  In1 : Inport
  AddSub{,1..3,5..9,11..13} (12 alike) : xbsIndex_r4/AddSub  mode=Addition  use_carryin=off  use_carryout=off  en=off  latency=0  precision=User Defined  arith_type="Signed  (2's comp)"  n_bits=17  bin_pt=4  quantization=Truncate  overflow=Wrap  use_behavioral_HDL=off  hw_selection=Fabric  pipelined=off  dbl_ovrd=off  block_type=addsub
  AddSub10 : xbsIndex_r4/AddSub  mode=Addition  use_carryin=off  use_carryout=off  en=off  latency=0  precision=Full  arith_type="Signed  (2's comp)"  n_bits=18  bin_pt=4  quantization=Truncate  overflow=Wrap  use_behavioral_HDL=off  hw_selection=Fabric  pipelined=off  dbl_ovrd=off  block_type=addsub
  AddSub14 : xbsIndex_r4/AddSub  mode=Addition  use_carryin=off  use_carryout=off  en=off  latency=0  precision=Full  arith_type="Signed  (2's comp)"  n_bits=18  bin_pt=4  quantization=Truncate  overflow=Wrap  use_behavioral_HDL=off  hw_selection=Fabric  pipelined=off  dbl_ovrd=off  block_type=addsub
  AddSub4 : xbsIndex_r4/AddSub  mode=Addition  use_carryin=off  use_carryout=off  en=off  latency=0  precision=Full  arith_type="Signed  (2's comp)"  n_bits=18  bin_pt=4  quantization=Truncate  overflow=Wrap  use_behavioral_HDL=off  hw_selection=Fabric  pipelined=off  dbl_ovrd=off  block_type=addsub
  Delay1 : xbsIndex_r4/Delay  rst=off  infoeditControl=Selection of Reset will increase slice count due to use of real FFs and instead of SRLs  en=off  latency=1  reg_retiming=off  dbl_ovrd=off  block_type=delay
  Delay10 : xbsIndex_r4/Delay  rst=off  infoeditControl=Selection of Reset will increase slice count due to use of real FFs and instead of SRLs  en=off  latency=7  reg_retiming=off  dbl_ovrd=off  block_type=delay
  Delay11 : xbsIndex_r4/Delay  rst=off  infoeditControl=Selection of Reset will increase slice count due to use of real FFs and instead of SRLs  en=off  latency=11  reg_retiming=off  dbl_ovrd=off  block_type=delay
  Delay12 : xbsIndex_r4/Delay  rst=off  infoeditControl=Selection of Reset will increase slice count due to use of real FFs and instead of SRLs  en=off  latency=12  reg_retiming=off  dbl_ovrd=off  block_type=delay
  Delay13 : xbsIndex_r4/Delay  rst=off  infoeditControl=Selection of Reset will increase slice count due to use of real FFs and instead of SRLs  en=off  latency=13  reg_retiming=off  dbl_ovrd=off  block_type=delay
  Delay14 : xbsIndex_r4/Delay  rst=off  infoeditControl=Selection of Reset will increase slice count due to use of real FFs and instead of SRLs  en=off  latency=14  reg_retiming=off  dbl_ovrd=off  block_type=delay
  Delay15 : xbsIndex_r4/Delay  rst=off  infoeditControl=Selection of Reset will increase slice count due to use of real FFs and instead of SRLs  en=off  latency=8  reg_retiming=off  dbl_ovrd=off  block_type=delay
  Delay2 : xbsIndex_r4/Delay  rst=off  infoeditControl=Selection of Reset will increase slice count due to use of real FFs and instead of SRLs  en=off  latency=2  reg_retiming=off  dbl_ovrd=off  block_type=delay
  Delay3 : xbsIndex_r4/Delay  rst=off  infoeditControl=Selection of Reset will increase slice count due to use of real FFs and instead of SRLs  en=off  latency=9  reg_retiming=off  dbl_ovrd=off  block_type=delay
  Delay4 : xbsIndex_r4/Delay  rst=off  infoeditControl=Selection of Reset will increase slice count due to use of real FFs and instead of SRLs  en=off  latency=15  reg_retiming=off  dbl_ovrd=off  block_type=delay
  Delay5 : xbsIndex_r4/Delay  rst=off  infoeditControl=Selection of Reset will increase slice count due to use of real FFs and instead of SRLs  en=off  latency=3  reg_retiming=off  dbl_ovrd=off  block_type=delay
  Delay6 : xbsIndex_r4/Delay  rst=off  infoeditControl=Selection of Reset will increase slice count due to use of real FFs and instead of SRLs  en=off  latency=10  reg_retiming=off  dbl_ovrd=off  block_type=delay
  Delay7 : xbsIndex_r4/Delay  rst=off  infoeditControl=Selection of Reset will increase slice count due to use of real FFs and instead of SRLs  en=off  latency=4  reg_retiming=off  dbl_ovrd=off  block_type=delay
  Delay8 : xbsIndex_r4/Delay  rst=off  infoeditControl=Selection of Reset will increase slice count due to use of real FFs and instead of SRLs  en=off  latency=5  reg_retiming=off  dbl_ovrd=off  block_type=delay
  Delay9 : xbsIndex_r4/Delay  rst=off  infoeditControl=Selection of Reset will increase slice count due to use of real FFs and instead of SRLs  en=off  latency=6  reg_retiming=off  dbl_ovrd=off  block_type=delay
  Out1 : Outport
  wires:
  AddSub/1 -> AddSub1/1
  AddSub9/1 -> AddSub12/2
  Delay1/1 -> AddSub/2
  Delay10/1 -> AddSub9/2
  Delay9/1 -> AddSub9/1
  Delay2/1 -> AddSub3/1
  Delay7/1 -> AddSub8/1
  AddSub1/1 -> AddSub4/1
  Delay8/1 -> AddSub8/2
  AddSub8/1 -> AddSub12/1
  Delay5/1 -> AddSub3/2
  AddSub3/1 -> AddSub1/2
  AddSub12/1 -> AddSub4/2
  AddSub6/1 -> AddSub10/2
  AddSub7/1 -> AddSub5/2
  Delay14/1 -> AddSub13/1
  AddSub13/1 -> AddSub6/2
  Delay11/1 -> AddSub7/2
  Delay13/1 -> AddSub11/2
  In1/1 -> AddSub/1, Delay4/1, Delay14/1, Delay13/1, Delay12/1, Delay11/1, Delay6/1, Delay3/1, Delay15/1, Delay10/1, Delay9/1, Delay8/1, Delay7/1, Delay5/1, Delay2/1, Delay1/1
  AddSub11/1 -> AddSub6/1
  AddSub5/1 -> AddSub10/1
  Delay6/1 -> AddSub7/1
  Delay3/1 -> AddSub2/2
  Delay12/1 -> AddSub11/1
  AddSub10/1 -> AddSub14/2
  AddSub2/1 -> AddSub5/1
  Delay4/1 -> AddSub13/2
  AddSub4/1 -> AddSub14/1
  AddSub14/1 -> Out1/1
  Delay15/1 -> AddSub2/1
